simulink model "Copy_of_linear_model"  (R2025a)
settings: Solver=VariableStepAuto  StartTime=0.0  StopTime=4  RelTol=1e-3
model workspace: external: MATLAB File C:\Users\Achref\Desktop\mecatro_mines_05\matlab\linear_model_constants.m (data not in the file)
values from neighbouring files (symbols this model uses):
  A_W = [0 1 0 ... (first row only)    [linear_model_constants.m]
  B_W = [-d_i 0 ... (first row only)    [linear_model_constants.m]
  C_W = [2/rho 0 -2]    [linear_model_constants.m]
  L = place(A_W', C_W', p_L)'    [linear_model_constants.m]
undefined symbols (not defined in the file or in its folder): A_XW, B_XW
settings Model: Creator=josep  LastModifiedBy=Achref

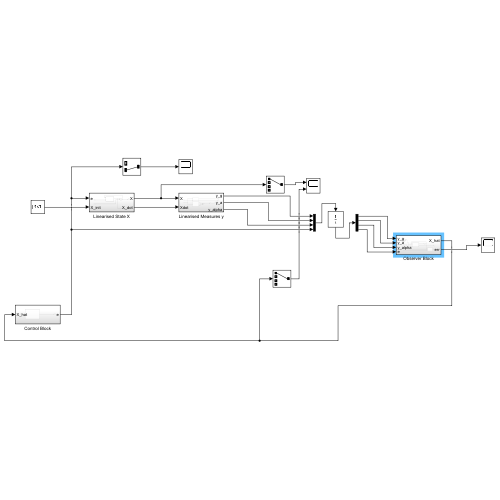
[thumbnail: Simulink's stored preview of the top-level diagram]
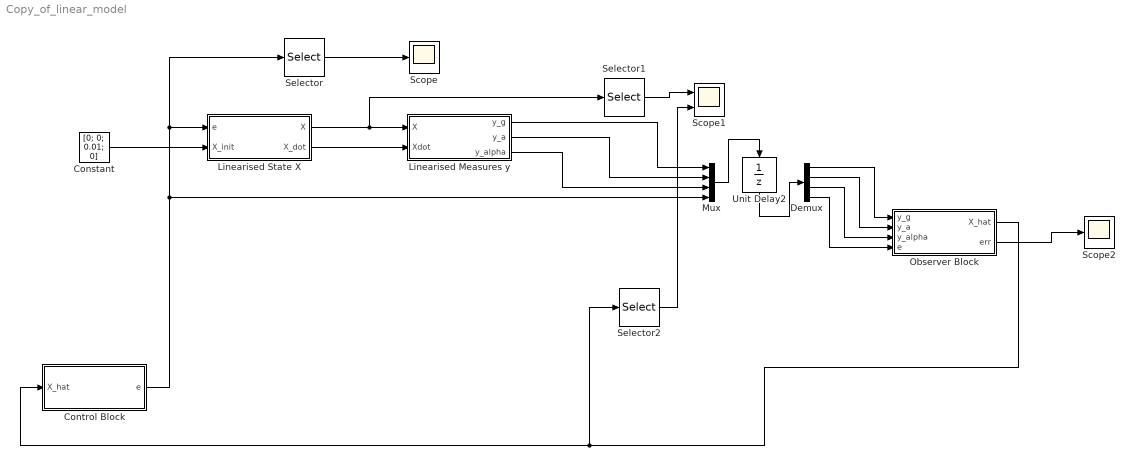
== system Copy_of_linear_model ==
  Constant : Constant  Value=[0; 0; 0.01; 0]
  Control Block : Subsystem
  Demux : Demux
  Linearised Measures y : Subsystem
  Linearised State X : Subsystem
  Mux : Mux
  Observer Block : Subsystem
  Scope : Scope
      settings: ActiveDisplayYMinimum=2.1477895791810231  ActiveDisplayYMaximum=2.8423079174060546
  Scope1 : Scope  NumInputPorts=2
      settings: ActiveDisplayYMinimum=-0.74568504293663151  ActiveDisplayYMaximum=2.0098142279473761
  Scope2 : Scope
      settings: ActiveDisplayYMinimum=-6.620114059536216  ActiveDisplayYMaximum=59.971823024951711  DataLoggingVariableName=ScopeData2
  Selector : Selector  InputPortWidth=2  IndexOptions=Index vector (dialog)  Indices=2  OutputSizes=1  RuntimeRangeChecks=on
  Selector1 : Selector  InputPortWidth=4  IndexOptions=Index vector (dialog)  Indices=1  OutputSizes=1  RuntimeRangeChecks=on
  Selector2 : Selector  InputPortWidth=4  IndexOptions=Index vector (dialog)  Indices=1  OutputSizes=1  RuntimeRangeChecks=on
  Unit Delay2 : UnitDelay  SampleTime=0.005  HasFrameUpgradeWarning=on
  wires:
  Linearised Measures y/1(y_g) -> Mux/1
  Linearised Measures y/3(y_alpha) -> Mux/3
  Linearised Measures y/2(y_a) -> Mux/2
  Linearised State X/2(X_dot) -> Linearised Measures y/2(Xdot)
  Control Block/1(e) -> Linearised State X/1(e), Selector/1, Mux/4
  Constant/1 -> Linearised State X/2(X_init)
  Linearised State X/1(X) -> Selector1/1, Linearised Measures y/1(X)
  Selector/1 -> Scope/1
  Observer Block/1(X_hat) -> Selector2/1, Control Block/1(X_hat)
  Selector1/1 -> Scope1/1
  Observer Block/2(err) -> Scope2/1
  Mux/1 -> Unit Delay2/1
  Unit Delay2/1 -> Demux/1
  Demux/1 -> Observer Block/1(y_g)
  Demux/2 -> Observer Block/2(y_a)
  Demux/3 -> Observer Block/3(y_alpha)
  Demux/4 -> Observer Block/4(e)
  Selector2/1 -> Scope1/2

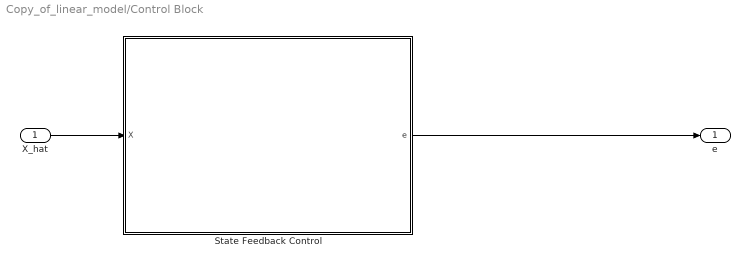
== system Copy_of_linear_model/Control Block ==
  X_hat : Inport  PortDimensions=4
  State Feedback Control : MATLAB Function  TreatAsAtomicUnit=on
  e : Outport  PortDimensions=2
  wires:
  X_hat/1 -> State Feedback Control/1(X)
  State Feedback Control/1(e) -> e/1

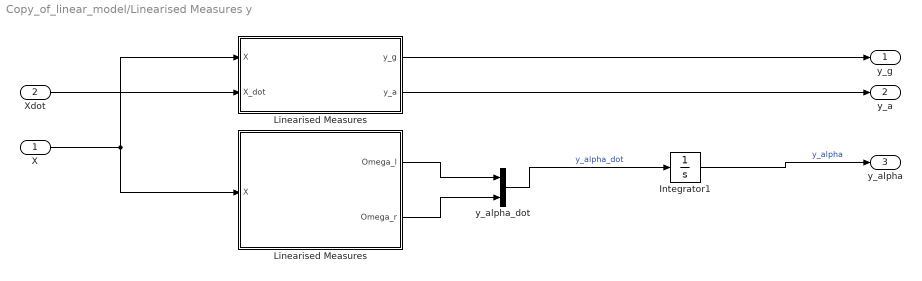
== system Copy_of_linear_model/Linearised Measures y ==
  X : Inport  PortDimensions=4
  Xdot : Inport  Port=2
  Integrator1 : Integrator
  Linearised Measures : MATLAB Function  TreatAsAtomicUnit=on
  "Linearised Measures " : MATLAB Function  TreatAsAtomicUnit=on
  y_alpha_dot : Mux  Inputs=2
  y_g : Outport
  y_a : Outport  Port=2
  y_alpha : Outport  Port=3
  wires:
  X/1 -> Linearised Measures/1(X), "Linearised Measures "/1(X)
  "Linearised Measures "/2(Omega_r) -> y_alpha_dot/2
  "Linearised Measures "/1(Omega_l) -> y_alpha_dot/1
  Linearised Measures/2(y_a) -> y_a/1
  Linearised Measures/1(y_g) -> y_g/1
  y_alpha_dot/1 -> Integrator1/1  "y_alpha_dot"
  Integrator1/1 -> y_alpha/1  "y_alpha"
  Xdot/1 -> Linearised Measures/2(X_dot)

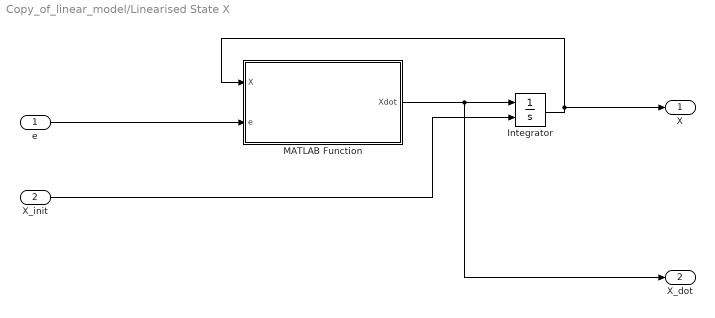
== system Copy_of_linear_model/Linearised State X ==
  e : Inport  PortDimensions=2
  X_init : Inport  Port=2  PortDimensions=4
  Integrator : Integrator  InitialConditionSource=external  InitialCondition=[0;0;0.5;0]
  MATLAB Function : MATLAB Function  TreatAsAtomicUnit=on
  X : Outport  PortDimensions=4
  X_dot : Outport  Port=2  PortDimensions=4
  wires:
  e/1 -> MATLAB Function/2(e)
  Integrator/1 -> MATLAB Function/1(X), X/1
  MATLAB Function/1(Xdot) -> X_dot/1, Integrator/1
  X_init/1 -> Integrator/2

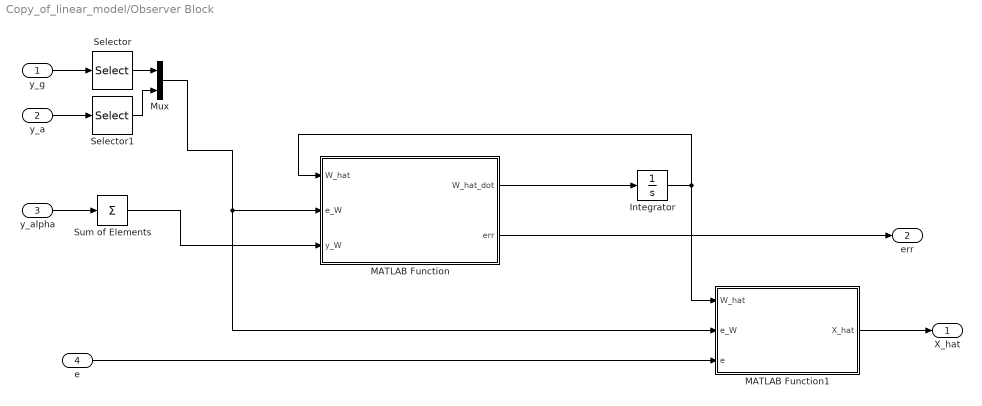
== system Copy_of_linear_model/Observer Block ==
  y_g : Inport  PortDimensions=3
  y_a : Inport  Port=2
  y_alpha : Inport  Port=3  PortDimensions=2
  e : Inport  Port=4  PortDimensions=2
  Integrator : Integrator
  MATLAB Function : MATLAB Function  TreatAsAtomicUnit=on
  MATLAB Function1 : MATLAB Function  TreatAsAtomicUnit=on
  Mux : Mux  Inputs=2
  Selector : Selector  IndexMode=Zero-based  InputPortWidth=3  IndexOptions=Index vector (dialog)  Indices=1  OutputSizes=1
  Selector1 : Selector  IndexMode=Zero-based  InputPortWidth=3  IndexOptions=Index vector (dialog)  Indices=0  OutputSizes=1
  Sum of Elements : Sum  Inputs=+
  X_hat : Outport  PortDimensions=4
  err : Outport  Port=2  PortDimensions=1
  wires:
  y_a/1 -> Selector1/1
  y_alpha/1 -> Sum of Elements/1
  MATLAB Function/1(W_hat_dot) -> Integrator/1
  Integrator/1 -> MATLAB Function/1(W_hat), MATLAB Function1/1(W_hat)
  e/1 -> MATLAB Function1/3(e)
  MATLAB Function1/1(X_hat) -> X_hat/1
  y_g/1 -> Selector/1
  Selector/1 -> Mux/1
  Selector1/1 -> Mux/2
  Mux/1 -> MATLAB Function1/2(e_W), MATLAB Function/2(e_W)
  Sum of Elements/1 -> MATLAB Function/3(y_W)
  MATLAB Function/2(err) -> err/1

== matlab function Copy_of_linear_model/Linearised Measures y/Linearised Measures ==
  data: X input; y_g output; y_a output; X_dot input
function [y_g, y_a] = lin_y(X, X_dot)

% y_g is the 3 dimensional output that is given by C_1 X + b_1
% y_a is the 3 dimensional output, that is given by C_2 X + b_2

theta     = X(1);
theta_dot = X(3);

u_dot      = X_dot(2);


% Gyroscope (body angular rates)
y_g = [0;
      theta_dot;
      0];

% Accelerometer (specific acceleration in IMU frame)
y_a = [u_dot * cos(theta) - g * sin(theta);
      0;
      u_dot * sin(theta) + g * cos(theta)];

== matlab function Copy_of_linear_model/Linearised State X/MATLAB Function ==
  data: X input; Xdot output; e input
function Xdot = nonlinmodel(X, e)

theta     = X(1);
u         = X(2);

theta_dot = X(3);

Ul = e(1);
Ur = e(2);



omega = u / Rho - theta_dot;

il = Ul/R - (k/R) * omega;
ir = Ur/R - (k/R) * omega;

tau_l = k * il;
tau_r = k * ir;




A11 = M + 2*Iw/rho^2;
A12 = mb*d * cos(theta);
A21 = mb*d * cos(theta);
A22 = Itoty + mb*d^2;

B1 = (1/rho)*(tau_l + tau_r) + mb*d*sin(theta)*theta_dot^2;
B2 = -(tau_l + tau_r) + mb*d*g*sin(theta);

A = [A11, A12; A21, A22];
B = [B1; B2];
sol = A\B;

u_dot       = sol(1);
theta_ddot  = sol(2);

Xdot = zeros(3,1);
Xdot(1) = theta_dot;
Xdot(2) = u_dot;
Xdot(3) = theta_ddot;
end

== matlab function Copy_of_linear_model/Linearised Measures y/Linearised Measures  ==
  data: X input; Omega_l output; Omega_r output
function [Omega_l, Omega_r] = lin_Omega(X)
theta_dot = X(3);
u=X(2);
Omega_l_r = 1/rho*u-theta_dot;
Omega_l = Omega_l_r;
Omega_r = Omega_l_r;

== matlab function Copy_of_linear_model/Observer Block/MATLAB Function ==
  data: W_hat input; e_W input; W_hat_dot output size=3; y_W input; L parameter; C_W parameter; A_W parameter; B_W parameter; err output
function [W_hat_dot, err] = observer(W_hat, e_W, y_W, L, C_W, A_W, B_W)

% Write the observer equation out, W_hat_dot = A * W_hat + B * e + L (y -
% y_hat) where e is a 2d vector as a linear combination of y_g and y_a

y_hat = C_W * W_hat;
W_hat_dot = A_W * W_hat + B_W * e_W + L * (y_W - y_hat);
err = norm(y_W - y_hat);

== matlab function Copy_of_linear_model/Observer Block/MATLAB Function1 ==
  data: W_hat input; e_W input; X_hat output; e input; A_XW parameter; B_XW parameter
function X_hat = W_hat_to_X_hat(W_hat, e_W, e, A_XW, B_XW)


X_hat = A_XW * W_hat + B_XW * e_W;

== matlab function Copy_of_linear_model/Control Block/State Feedback Control ==
  data: X input; e output; K parameter
function e = state_feedback(X, K)
    % Function that gives the control signal for the eqn
    % X_dot = (A - BK)X + Bkr, where u = -KX + r, where r is
    % a reference consant (or non constant maybe ?)
    
    % solving the system, we get that equilibrium will be reached at x_bar =
    % - (A - BK)^-1 Br, which means that if we set a reference r, we can control
    % where the system stabilises to. Thus, r = (K - B^-1 A)x_bar
    
    % the control signal "u" here is given by the sum of components of e, so e
    % should be 
    
     e_unlimited = -K * X;
     e = [min(max(e_unlimited(1), -12), 12)
          min(max(e_unlimited(2), -12), 12)];
     % e = -K * X;
end
